simulink model "VIDEO_SIM"  (R2022a)
settings: Solver=VariableStepAuto  StartTime=0.0  StopTime=350  RelTol=1e-3
libraries: uavsimlib x4
settings Model: PacingRate=3  Creator=trinc  LastModifiedBy=Aster

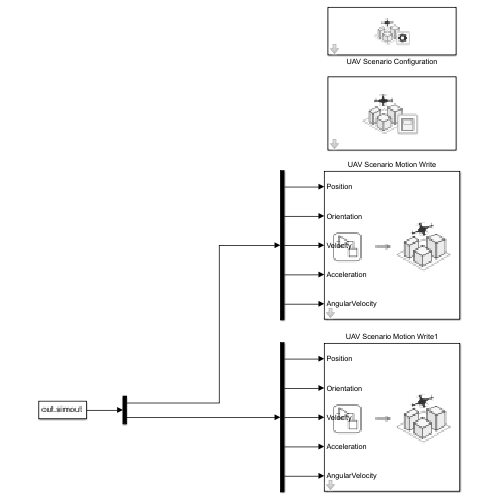
[thumbnail: Simulink's stored preview of the top-level diagram]
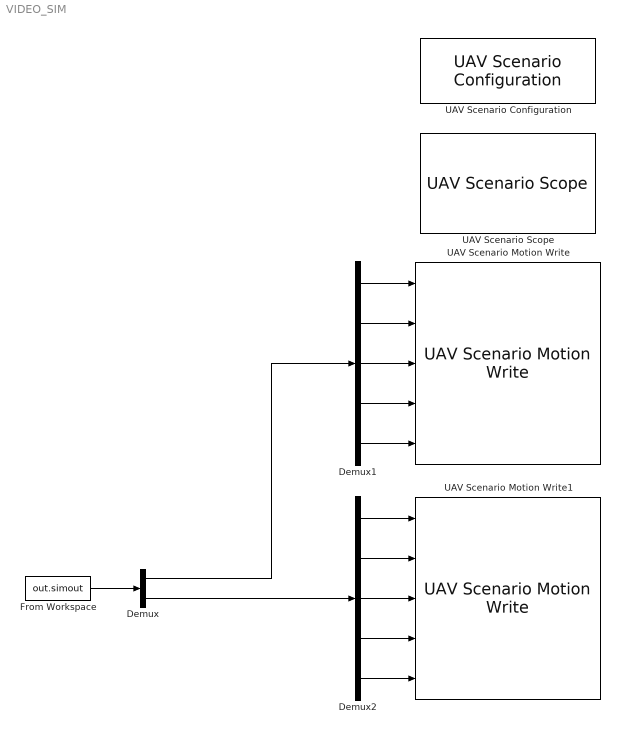
== system VIDEO_SIM ==
  Demux : Demux  Outputs=2
  Demux1 : Demux  Outputs=5
  Demux2 : Demux  Outputs=5
  From Workspace : FromWorkspace  VariableName=out.simout
  UAV Scenario Configuration : uavsimlib/UAV Scenario Configuration  Priority=-1  UAVScenarioObject=Scenario  SampleTime=0.1  UpdateParam=true  SensorMotionBusName='SensorMotionBus'  PlatformMotionBusName='PlatformMotionBus'  ScenarioMotionBusName='ScenarioMotionBus'  ScenarioMotionSignalName='ScenarioMotions'
      settings: SourceProductBaseCode=UV
  UAV Scenario Motion Write : uavsimlib/UAV Scenario Motion Write  Priority=0  PlatName='UAV'  ReferenceFrame=NED
      settings: SourceProductBaseCode=UV
  UAV Scenario Motion Write1 : uavsimlib/UAV Scenario Motion Write  Priority=0  PlatName='UAV2'  ReferenceFrame=NED
      settings: SourceProductBaseCode=UV
  UAV Scenario Scope : uavsimlib/UAV Scenario Scope  Priority=1  SensorNameTable={}  SampleTime=0.1
      settings: SourceProductBaseCode=UV
  wires:
  From Workspace/1 -> Demux/1
  Demux1/5 -> UAV Scenario Motion Write/5
  Demux1/4 -> UAV Scenario Motion Write/4
  Demux1/3 -> UAV Scenario Motion Write/3
  Demux1/2 -> UAV Scenario Motion Write/2
  Demux1/1 -> UAV Scenario Motion Write/1
  Demux2/3 -> UAV Scenario Motion Write1/3
  Demux2/2 -> UAV Scenario Motion Write1/2
  Demux2/4 -> UAV Scenario Motion Write1/4
  Demux2/5 -> UAV Scenario Motion Write1/5
  Demux2/1 -> UAV Scenario Motion Write1/1
  Demux/2 -> Demux2/1
  Demux/1 -> Demux1/1
